simulink model "control_pos_3dof_conMI"  (R2023b)
settings: Solver=ode45  StartTime=0.0  StopTime=tsim  FixedStep=tstep  MaxStep=tstep  RelTol=1e-3
undefined symbols (not defined in the file): a0, a1, MI_Contr1, MI_Contr2, MI_Contr3, MI_motor1, MI_motor2, MI_motor3, robot_params, sigbuilder_block, t_qeq_init, t_tr_init, tau_L
(part 4 of 4)

== matlab function control_pos_3dof_conMI/Controlador de posición/Modelo dinámico ==
  data: robot_params input; robot_din output Bus: robot_din_bus size=1; q input size=[3,1]; dq input size=[3,1]
function robot_din = fcn(robot_params,q,dq)

%d1 = robot_params.d(1);
l2 = robot_params.l(2);
lc2 = robot_params.lc(2);
%l3 = robot_params.l(3);
lc3 = robot_params.lc(3);

%m1 = robot_params.m(1);
m2 = robot_params.m(2);
m3 = robot_params.m(3);

Iz1 = robot_params.I(1,3);
Iy2 = robot_params.I(2,2);
Iz2 = robot_params.I(2,3);
Iy3 = robot_params.I(3,2);
Iz3 = robot_params.I(3,3);

g = 9.81;

q1 = q(1);
q2 = q(2);
q3 = q(3);

dq1 = dq(1);
dq2 = dq(2);
dq3 = dq(3);

D = zeros(3,3);

D(1,1) = Iz1 + Iz2 + Iz3 + (m2/2)*lc2^2*(1+cos(2*q2)) ...
       + (m3/2)*(l2^2*(1+cos(2*q2)) + 2*l2*lc3*(cos(2*q2+q3)+cos(q3)) ...
       + lc3^2*(1+cos(2*q2+2*q3)));

D(2,2) = Iy2 + Iy3 + m2*lc2^2 + m3*(l2^2 + 2*l2*lc3*cos(q3) + lc3^2);
D(2,3) = Iy3 + m3*(l2*lc3*cos(q3) + lc3^2);

D(3,2) = Iy3 + m3*(l2*lc3*cos(q3) + lc3^2);
D(3,3) = Iy3 + m3*lc3^2;

C = zeros(3,3);

C(1,2) = - ((m2*lc2^2*sin(2*q2)) ...
         + m3*(l2^2*sin(2*q2) + 2*l2*lc3*sin(2*q2+q3) ...
         + lc3^2*sin(2*q2+2*q3)))*dq1;
C(1,3) = - m3*(l2*lc3*(sin(2*q2+q3)+sin(q3)) ...
         + lc3^2*(sin(2*q2+2*q3)))*dq1;

C(2,1) =   ((m2/2)*(lc2^2*sin(2*q2)) ...
         + (m3/2)*(l2^2*sin(2*q2) + 2*l2*lc3*sin(2*q2+q3) ...
         + lc3^2*sin(2*q2+2*q3)))*dq1;
C(2,2) = - 2*m3*l2*lc3*sin(q3)*dq3;
C(2,3) = - m3*l2*lc3*sin(q3)*dq3;

C(3,1) =   (m3/2)*(l2*lc3*(sin(2*q2+q3) + sin(q3)) ...
         + lc3^2*sin(2*q2+2*q3))*dq1;
C(3,2) =   m3*l2*lc3*sin(q3)*dq2;

G = zeros(3,1);

G(2,1) = m2*lc2*cos(q2) + m3*(l2*cos(q2) + lc3*cos(q2+q3));
G(3,1) = m3*lc3*cos(q2+q3);


robot_din = struct('D',D,'C',C,'G',G,'g',9.81);

%busInfo = Simulink.Bus.createObject(robot_dyn);

== matlab function control_pos_3dof_conMI/Dinámica inversa (referencia)/Dinamica inversa (referencia) ==
  data: robot_params input; q input size=[3,1]; tau_s output size=[3,1]; dq input size=[3,1]; ddq input size=[3,1]
function tau_s = dyn_inv(robot_params,q,dq,ddq)

%d1 = robot_params.d(1);
l2 = robot_params.l(2);
lc2 = robot_params.lc(2);
%l3 = robot_params.l(3);
lc3 = robot_params.lc(3);

%m1 = robot_params.m(1);
m2 = robot_params.m(2);
m3 = robot_params.m(3);

Iz1 = robot_params.I(1,3);
Iy2 = robot_params.I(2,2);
Iz2 = robot_params.I(2,3);
Iy3 = robot_params.I(3,2);
Iz3 = robot_params.I(3,3);

g = 9.81;

q1 = q(1);
q2 = q(2);
q3 = q(3);

dq1 = dq(1);
dq2 = dq(2);
dq3 = dq(3);

D = zeros(3,3);

D(1,1) = Iz1 + Iz2 + Iz3 + (m2/2)*lc2^2*(1+cos(2*q2)) ...
       + (m3/2)*(l2^2*(1+cos(2*q2)) + 2*l2*lc3*(cos(2*q2+q3)+cos(q3)) ...
       + lc3^2*(1+cos(2*q2+2*q3)));

D(2,2) = Iy2 + Iy3 + m2*lc2^2 + m3*(l2^2 + 2*l2*lc3*cos(q3) + lc3^2);
D(2,3) = Iy3 + m3*(l2*lc3*cos(q3) + lc3^2);

D(3,2) = Iy3 + m3*(l2*lc3*cos(q3) + lc3^2);
D(3,3) = Iy3 + m3*lc3^2;

C = zeros(3,3);

C(1,2) = - ((m2*lc2^2*sin(2*q2)) ...
         + m3*(l2^2*sin(2*q2) + 2*l2*lc3*sin(2*q2+q3) ...
         + lc3^2*sin(2*q2+2*q3)))*dq1;
C(1,3) = - m3*(l2*lc3*(sin(2*q2+q3)+sin(q3)) ...
         + lc3^2*(sin(2*q2+2*q3)))*dq1;

C(2,1) =   ((m2/2)*(lc2^2*sin(2*q2)) ...
         + (m3/2)*(l2^2*sin(2*q2) + 2*l2*lc3*sin(2*q2+q3) ...
         + lc3^2*sin(2*q2+2*q3)))*dq1;
C(2,2) = - 2*m3*l2*lc3*sin(q3)*dq3;
C(2,3) = - m3*l2*lc3*sin(q3)*dq3;

C(3,1) =   (m3/2)*(l2*lc3*(sin(2*q2+q3) + sin(q3)) ...
         + lc3^2*sin(2*q2+2*q3))*dq1;
C(3,2) =   m3*l2*lc3*sin(q3)*dq2;

G = zeros(3,1);

G(2,1) = m2*lc2*cos(q2) + m3*(l2*cos(q2) + lc3*cos(q2+q3));
G(3,1) = m3*lc3*cos(q2+q3);


tau_s = D*ddq + C*dq + G*g;

== matlab function control_pos_3dof_conMI/Modelo robot manipulador (Dinámica directa)/Dinámica directa(1) ==
  data: robot_params input; q input size=[3,1]; ddq output size=[3,1]; dq input size=[3,1]; tau_R input size=[3,1]; tau_L input size=[3,1]
function ddq = fcn(robot_params,q,dq,tau_R,tau_L)

%d1 = robot_params.d(1);
l2 = robot_params.l(2);
lc2 = robot_params.lc(2);
%l3 = robot_params.l(3);
lc3 = robot_params.lc(3);

%m1 = robot_params.m(1);
m2 = robot_params.m(2);
m3 = robot_params.m(3);

Iz1 = robot_params.I(1,3);
Iy2 = robot_params.I(2,2);
Iz2 = robot_params.I(2,3);
Iy3 = robot_params.I(3,2);
Iz3 = robot_params.I(3,3);

g = 9.81;

q1 = q(1);
q2 = q(2);
q3 = q(3);

dq1 = dq(1);
dq2 = dq(2);
dq3 = dq(3);

D = zeros(3,3);

D(1,1) = Iz1 + Iz2 + Iz3 + (m2/2)*lc2^2*(1+cos(2*q2)) ...
       + (m3/2)*(l2^2*(1+cos(2*q2)) + 2*l2*lc3*(cos(2*q2+q3)+cos(q3)) ...
       + lc3^2*(1+cos(2*q2+2*q3)));

D(2,2) = Iy2 + Iy3 + m2*lc2^2 + m3*(l2^2 + 2*l2*lc3*cos(q3) + lc3^2);
D(2,3) = Iy3 + m3*(l2*lc3*cos(q3) + lc3^2);

D(3,2) = Iy3 + m3*(l2*lc3*cos(q3) + lc3^2);
D(3,3) = Iy3 + m3*lc3^2;

C = zeros(3,3);

C(1,2) = - ((m2*lc2^2*sin(2*q2)) ...
         + m3*(l2^2*sin(2*q2) + 2*l2*lc3*sin(2*q2+q3) ...
         + lc3^2*sin(2*q2+2*q3)))*dq1;
C(1,3) = - m3*(l2*lc3*(sin(2*q2+q3)+sin(q3)) ...
         + lc3^2*(sin(2*q2+2*q3)))*dq1;

C(2,1) =   ((m2/2)*(lc2^2*sin(2*q2)) ...
         + (m3/2)*(l2^2*sin(2*q2) + 2*l2*lc3*sin(2*q2+q3) ...
         + lc3^2*sin(2*q2+2*q3)))*dq1;
C(2,2) = - 2*m3*l2*lc3*sin(q3)*dq3;
C(2,3) = - m3*l2*lc3*sin(q3)*dq3;

C(3,1) =   (m3/2)*(l2*lc3*(sin(2*q2+q3) + sin(q3)) ...
         + lc3^2*sin(2*q2+2*q3))*dq1;
C(3,2) =   m3*l2*lc3*sin(q3)*dq2;

G = zeros(3,1);

G(2,1) = m2*lc2*cos(q2) + m3*(l2*cos(q2) + lc3*cos(q2+q3));
G(3,1) = m3*lc3*cos(q2+q3);



ddq = D^-1*(-C*dq-G*g+(tau_R-tau_L));
